simulink model "LQR_6DoF_v4"  (R2022b)
settings: Solver=ode45  StartTime=0.0  StopTime=10  FixedStep=0.01  RelTol=1e-3
undefined symbols (not defined in the file): beta, e0_0, e1_0, e2_0, e3_0, eul0, G0, gamma, gc, geometry, Js, Js0, K_lqrq, m_dry, m_fuel, m_full, m_max, mass, omega0, parameters, pos0, r_cg, rcgs, ref_eul, Tensors, vel0, xq0
libraries: sharedtransform x38, simulink_extras x21, matrix_library x12, sharedutil x4, aerolibpropulsion2 x1
(part 1 of 2)
settings Model: Creator=User  LastModifiedBy=User
settings SolverCC: MaxConsecutiveMinStep=10

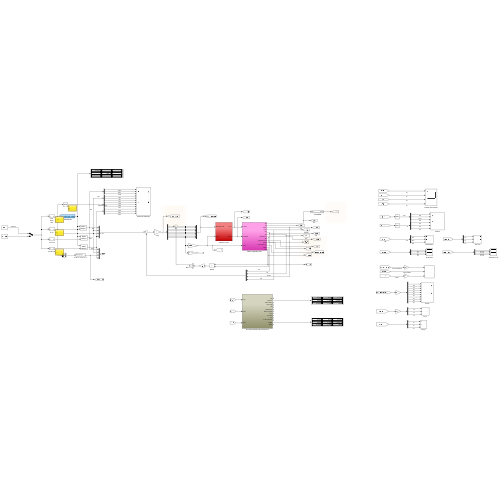
[thumbnail: Simulink's stored preview of the top-level diagram]
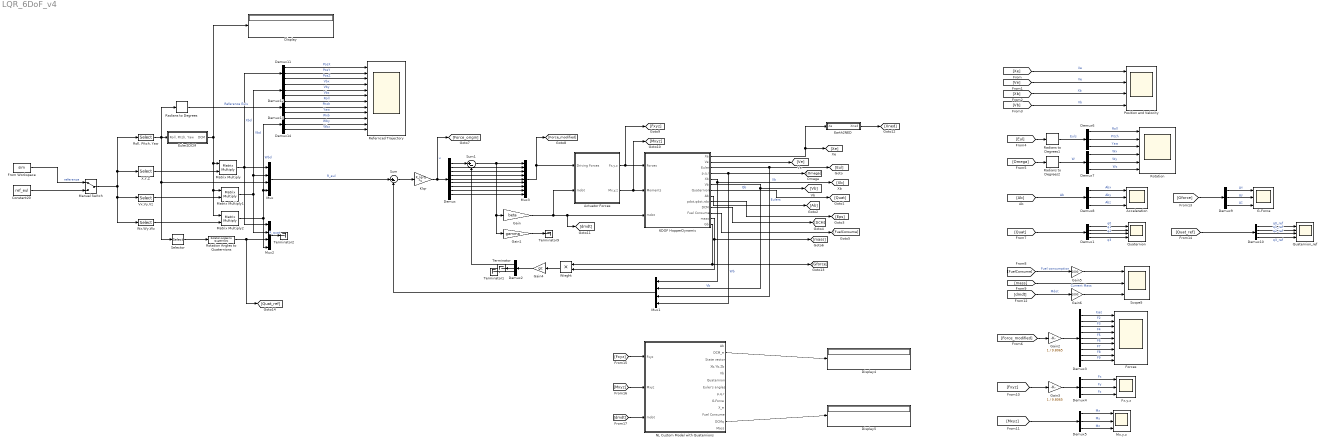
== system LQR_6DoF_v4 ==
  6DOF HopperDynamic : Subsystem
  Acceleration : Scope  NumInputPorts=3
  Actuator Forces : Subsystem
  Constant20 : Constant  Value=ref_eul
  Demux : Demux  Outputs=9
  Demux1 : Demux
  Demux10 : Demux
  Demux{2,4..9,11..14} (11 alike) : Demux  Outputs=3
  Demux3 : Demux  Outputs=9
  Display : Display
  Display4 : Display
  Display5 : Display
  Earth2NED : Subsystem
  Euler2DCM : Subsystem
  Forces : Scope  NumInputPorts=9
  From Workspace : FromWorkspace  VariableName=sim
  Fx,y,z : Scope  NumInputPorts=3
  G-Force : Scope  NumInputPorts=3
  Gain : Gain  Gain=beta
  Gain1 : Gain  Gain=gamma
  Gain2 : Gain  Gain=1 / 9.8065
  Gain3 : Gain  Gain=1 / 9.8065
  Gain4 : Gain  Gain=gc
  Gain5 : Gain  Gain=1000
  Gain6 : Gain  Gain=1000
  Klqr : Gain  Gain=K_lqrq  Multiplication=Matrix(K*u)
  Manual Switch : ManualSwitch
  Matrix Multiply : Product  Multiplication=Matrix(*)
  Matrix Multiply1 : Product  Multiplication=Matrix(*)
  Matrix Multiply2 : Product  Multiplication=Matrix(*)
  Mux : Mux
  Mux1 : Mux
  Mux2 : Mux
  Mux3 : Mux  Inputs=9
  Mx,y,z : Scope  NumInputPorts=3
  NL Custom Model with Quaternions : Subsystem
  Position and Velocity : Scope  NumInputPorts=4
  Quaternion : Scope  NumInputPorts=4
  Quaternion_ref : Scope  NumInputPorts=4
  Radians to Degrees : simulink_extras/Transformations/Radians to Degrees
  Radians to Degrees1 : simulink_extras/Transformations/Radians to Degrees
  Radians to Degrees2 : simulink_extras/Transformations/Radians to Degrees
  Refernced Trajectory : Scope  NumInputPorts=12
  "Roll, Pitch, Yaw" : Selector  InputPortWidth=12  IndexOptions=Index vector (dialog)  Indices=[7:9]  OutputSizes=1
  Rotation : Scope  NumInputPorts=6
  Rotation Angles to Quaternions : sharedtransform/Rotation Angles to Quaternions  rotationOrder=ZYX  aMode=aMode
  Scope5 : Scope  NumInputPorts=3
  Selector : Selector  InputPortWidth=3  IndexOptions=Index vector (dialog)  Indices=[2 3 1]  OutputSizes=1
  Sum : Sum  Inputs=|+-
  Sum1 : Sum  Inputs=|+-
  Terminator{,1..2,9} (4 alike) : Terminator
  Vx,Vy,Vz : Selector  InputPortWidth=12  IndexOptions=Index vector (dialog)  Indices=[4:6]  OutputSizes=1
  Wieght : Product
  Wx,Wy,Wz : Selector  InputPortWidth=12  IndexOptions=Index vector (dialog)  Indices=[10:12]  OutputSizes=1
  X,Y,Z : Selector  InputPortWidth=12  IndexOptions=Index vector (dialog)  Indices=[1:3]  OutputSizes=1
  wires:
  Constant20/1 -> Manual Switch/2
  From Workspace/1 -> Manual Switch/1  "reference"
  "Roll, Pitch, Yaw"/1 -> Radians to Degrees/1, Euler2DCM/1("Roll, Pitch, Yaw"), Selector/1, Mux/3
  Manual Switch/1 -> Wx,Wy,Wz/1, Vx,Vy,Vz/1, X,Y,Z/1, "Roll, Pitch, Yaw"/1
  Euler2DCM/1(DCM) -> Display/1, Matrix Multiply2/1, Matrix Multiply1/1, Matrix Multiply/1
  Klqr/1 -> [Force_origin], Demux/1  "u"
  X,Y,Z/1 -> Matrix Multiply/2
  Vx,Vy,Vz/1 -> Matrix Multiply1/2
  Wx,Wy,Wz/1 -> Matrix Multiply2/2
  Matrix Multiply/1 -> Demux11/1, Mux2/1, Mux/1  "Xbd"
  Actuator Forces/1(Fx,y,z) -> [Fxyz], 6DOF HopperDynamic/1(Forces)
  Actuator Forces/2(Mx,y,z) -> [Mxyz], 6DOF HopperDynamic/2(Moments)
  Demux/1 -> Sum1/1
  Demux/2 -> Mux3/2
  Demux/4 -> Mux3/4
  Demux/6 -> Mux3/6
  Demux/8 -> Mux3/8
  Gain/1 -> Actuator Forces/2(mdot), [dmdt], 6DOF HopperDynamic/3(mdot)
  Gain1/1 -> Terminator9/1
  Matrix Multiply1/1 -> Mux2/2, Demux12/1, Mux/2  "Vbd"
  Matrix Multiply2/1 -> Demux14/1, Mux/4, Mux2/4  "Wbd"
  Radians to Degrees/1 -> Demux13/1  "Reference Euls"
  6DOF HopperDynamic/1(Xe) -> Earth2NED/1(Xe), [Xe]
  6DOF HopperDynamic/2(Ve) -> [Ve]
  6DOF HopperDynamic/3(Euler) -> Mux1/3, [Eul]  "Eulers"
  6DOF HopperDynamic/4(p,q,r) -> Mux1/4, [Omega]  "Wb"
  6DOF HopperDynamic/5(Xb) -> [Xb], Mux1/1  "Xb"
  6DOF HopperDynamic/6(Vb) -> Mux1/2, [Vb]  "Vb"
  6DOF HopperDynamic/7(Quaternion) -> [Quat]  "Qb"
  6DOF HopperDynamic/8(Ab) -> [Ab]
  6DOF HopperDynamic/9(pdot,qdot,rdot) -> [Eps]
  6DOF HopperDynamic/10(DCM) -> [DCM]
  6DOF HopperDynamic/11(Fuel Consume) -> [FuelConsume]
  6DOF HopperDynamic/12(mass) -> Wieght/2, [mass]
  Selector/1 -> Rotation Angles to Quaternions/1
  Rotation Angles to Quaternions/1 -> [Quat_ref], Mux2/3
  Mux/1 -> Sum/1  "R_eul"
  Sum/1 -> Klqr/1
  Mux1/1 -> Sum/2
  [Xe] -> Position and Velocity/1  "Xe"
  [Ve] -> Position and Velocity/2  "Ve"
  [Xb] -> Position and Velocity/3  "Xb"
  [Vb] -> Position and Velocity/4  "Vb"
  [Eul] -> Radians to Degrees1/1
  [Omega] -> Radians to Degrees2/1
  Radians to Degrees1/1 -> Demux6/1  "Euls"
  Radians to Degrees2/1 -> Demux7/1  "W"
  [Ab] -> Demux8/1  "Ab"
  [Quat] -> Demux1/1
  Demux1/1 -> Quaternion/1  "q0"
  Demux1/2 -> Quaternion/2  "q1"
  Demux1/3 -> Quaternion/3  "q2"
  Demux1/4 -> Quaternion/4  "q3"
  [FuelConsume] -> Gain5/1  "Fuel consumption"
  [mass] -> Scope5/2  "Current Mass"
  Demux/3 -> Mux3/3
  Demux/5 -> Mux3/5
  Demux/7 -> Mux3/7
  Demux/9 -> Mux3/9
  Sum1/1 -> Gain1/1, Gain/1, Mux3/1
  Mux3/1 -> [Force_modified], Actuator Forces/1(Driving Forces)
  6DOF HopperDynamic/13(Gb) -> [Gforce], Wieght/1
  Wieght/1 -> Gain4/1
  Demux2/1 -> Sum1/2
  Demux2/2 -> Terminator/1
  Demux2/3 -> Terminator1/1
  [Force_modified] -> Gain2/1
  Gain2/1 -> Demux3/1
  Demux3/1 -> Forces/1  "Fjet"
  Demux3/2 -> Forces/2  "F2"
  Demux3/3 -> Forces/3  "F3"
  Demux3/4 -> Forces/4  "F4"
  Demux3/5 -> Forces/5  "F5"
  Demux3/6 -> Forces/6  "F6"
  Demux3/7 -> Forces/7  "F7"
  Demux3/8 -> Forces/8  "F8"
  Demux3/9 -> Forces/9  "F9"
  [Fxyz] -> Gain3/1
  Gain3/1 -> Demux4/1
  Demux4/1 -> Fx,y,z/1  "Fx"
  Demux4/2 -> Fx,y,z/2  "Fy"
  Demux4/3 -> Fx,y,z/3  "Fz"
  Demux5/2 -> Mx,y,z/2  "My"
  Demux5/1 -> Mx,y,z/1  "Mx"
  [Mxyz] -> Demux5/1
  Demux5/3 -> Mx,y,z/3  "Mz"
  Demux6/2 -> Rotation/2  "Pitch"
  Demux6/1 -> Rotation/1  "Roll"
  Demux6/3 -> Rotation/3  "Yaw"
  Demux7/1 -> Rotation/4  "Wx"
  Demux7/2 -> Rotation/5  "Wy"
  Demux7/3 -> Rotation/6  "Wz"
  Demux8/1 -> Acceleration/1  "Abx"
  Demux8/2 -> Acceleration/2  "Aby"
  Demux8/3 -> Acceleration/3  "Abz"
  [dmdt] -> Gain6/1  "Mdot"
  Earth2NED/1(Xned) -> [Xned]
  [Gforce] -> Demux9/1
  Demux9/1 -> G-Force/1  "gx"
  Demux9/2 -> G-Force/2  "gy"
  Demux9/3 -> G-Force/3  "gz"
  Demux10/2 -> Quaternion_ref/2  "q1_ref"
  Demux10/4 -> Quaternion_ref/4  "q3_ref"
  Demux10/1 -> Quaternion_ref/1  "q0_ref"
  Demux10/3 -> Quaternion_ref/3  "q2_ref"
  [Quat_ref] -> Demux10/1
  [Fxyz] -> NL Custom Model with Quaternions/1(Fxyz)
  [Mxyz] -> NL Custom Model with Quaternions/2(Mxyz)
  [dmdt] -> NL Custom Model with Quaternions/3(mdot)
  NL Custom Model with Quaternions/2(DCM_e) -> Display4/1
  NL Custom Model with Quaternions/12(DCMq) -> Display5/1
  Mux2/1 -> Terminator2/1  "R_quat"
  Gain4/1 -> Demux2/1
  Gain5/1 -> Scope5/1
  Gain6/1 -> Scope5/3
  Demux11/1 -> Refernced Trajectory/1  "PosX"
  Demux11/2 -> Refernced Trajectory/2  "PosY"
  Demux11/3 -> Refernced Trajectory/3  "PosZ"
  Demux12/1 -> Refernced Trajectory/4  "Vbx"
  Demux12/2 -> Refernced Trajectory/5  "Vby"
  Demux12/3 -> Refernced Trajectory/6  "Vbz"
  Demux13/1 -> Refernced Trajectory/7  "Roll"
  Demux13/2 -> Refernced Trajectory/8  "Pitch"
  Demux13/3 -> Refernced Trajectory/9  "Yaw"
  Demux14/1 -> Refernced Trajectory/10  "Wxb"
  Demux14/2 -> Refernced Trajectory/11  "Wby"
  Demux14/3 -> Refernced Trajectory/12  "Wbz"

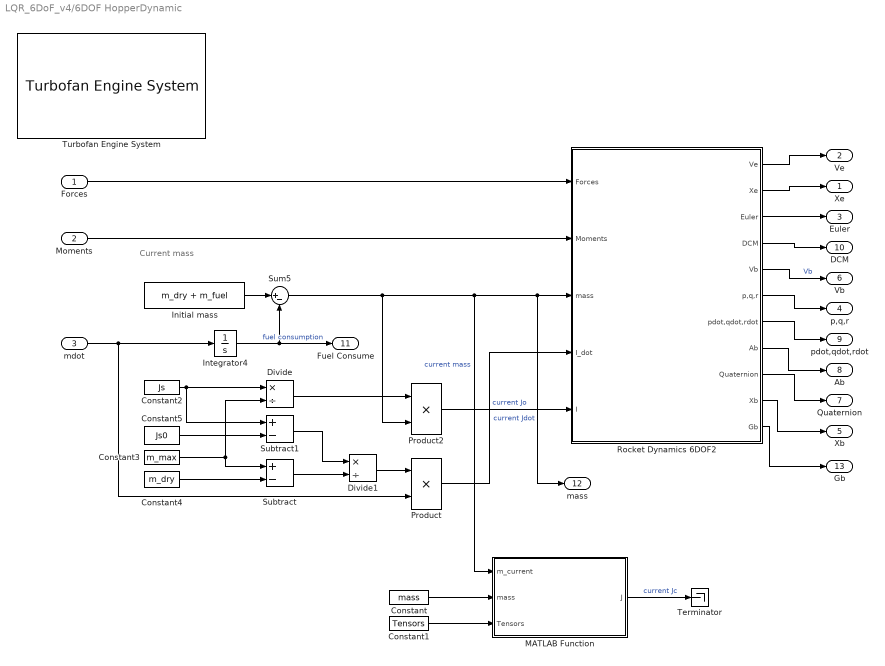
== system LQR_6DoF_v4/6DOF HopperDynamic ==
  note: Current mass
  Forces : Inport
  Moments : Inport  Port=2
  mdot : Inport  Port=3
  Constant : Constant  Value=mass
  Constant1 : Constant  Value=Tensors
  Constant2 : Constant  Value=Js
  Constant3 : Constant  Value=m_max
  Constant4 : Constant  Value=m_dry
  Constant5 : Constant  Value=Js0
  Divide : Product  Inputs=*/
  Divide1 : Product  Inputs=*/
  Initial mass : Constant  Value=m_dry + m_fuel
  Integrator4 : Integrator
  MATLAB Function : MATLAB Function  TreatAsAtomicUnit=on
  Product : Product  SaturateOnIntegerOverflow=on  OutDataTypeStr=Inherit: Same as first input
  Product2 : Product  SaturateOnIntegerOverflow=on  OutDataTypeStr=Inherit: Same as first input
  Rocket Dynamics 6DOF2 : Subsystem  mask(6DOF EoM (Body Axis)){xme_0=pos0', Vm_0=vel0', eul_0=eul0', pm_0=omega0', k_quat=1.0, xme_statename='', Vm_statename='', quat_statename='', pm_statename=''}
      mask prompts: xme_0 "Initial position in inertial axes [Xe,Ye,Ze]:"; Vm_0 "Initial velocity in body axes [U,v,w]:"; eul_0 "Initial Euler orientation [roll, pitch, yaw]:"; pm_0 "Initial body rotation rates [p,q,r]:"; k_quat "Gain for quaternion normalization:"; xme_statename "Position: e.g., {'Xe', 'Ye', 'Ze'}"; Vm_statename "Velocity: e.g., {'U', 'v', 'w'}"; quat_statename "Quaternion vector: e.g., {'qr', 'qi', 'qj', 'qk'}"; pm_statename "Body rotation rates: e.g., {'p', 'q', 'r'}"
      mask help: Integrate the six-degress-of-freedom equations of motion in body axes
      mask DialogControl Container8 Prompt: Main
      mask DialogControl Container9 Prompt: State Attributes
      mask DialogControl Container10 Prompt: State Names
      mask Display:
      | port_label('input',1,'F_{xyz}(N)','texmode','on');
      | port_label('input',2,'M_{xyz}(N\cdotm)','texmode','on');
      | port_label('input',3,'m (kg)','texmode','on');
      | port_label('input',4,'dI/dt (kg\cdotm^2/s)','texmode','on');
      | port_label('input',5,'I (kg\cdotm^2)','texmode','on');
      | port_label('output',1,'V_e (m/s)','texmode','on');
      | port_label('output',2,'X_e (m)','texmode','on');
      | port_label('output',3,'\phi \theta \psi (rad)','texmode','on');
      | port_label('output',4,'DCM_{be}','texmode','on');
      | port_label('output',5,'V_b (m/s)','texmode','on');
      | port_label('output',6,'\omega_b (rad/s)','texmode','on');
      | port_label('output',7,'d\omega_b/dt (rad/s^2)','texmode','on');
      | port_label('output',8,'A_{bb} (m/s^2)','texmode','on');
  Subtract : Sum  Inputs=+-
  Subtract1 : Sum  Inputs=+-
  Sum5 : Sum  Inputs=|+-
  Terminator : Terminator
  Turbofan Engine System : aerolibpropulsion2/Turbofan Engine System  units=Metric (MKS)  ic_source=Internal  IC=0  Fmax=45000  tau=1  SFC=0.35  Nt=0.9
  Xe : Outport
  Ve : Outport  Port=2
  Euler : Outport  Port=3
  p,q,r : Outport  Port=4
  Xb : Outport  Port=5
  Vb : Outport  Port=6
  Quaternion : Outport  Port=7
  Ab : Outport  Port=8
  pdot,qdot,rdot : Outport  Port=9
  DCM : Outport  Port=10
  Fuel Consume : Outport  Port=11
  mass : Outport  Port=12
  Gb : Outport  Port=13
  wires:
  Rocket Dynamics 6DOF2/6(p,q,r) -> p,q,r/1
  Divide/1 -> Product2/1
  Integrator4/1 -> Fuel Consume/1, Sum5/2  "fuel consumption"
  Constant3/1 -> Divide/2, Subtract/1
  Product2/1 -> Rocket Dynamics 6DOF2/5(I)  "current Jo"
  Rocket Dynamics 6DOF2/4(DCM) -> DCM/1
  Constant5/1 -> Subtract1/2
  Rocket Dynamics 6DOF2/5(Vb) -> Vb/1  "Vb"
  Subtract1/1 -> Divide1/1
  Divide1/1 -> Product/1
  mdot/1 -> Product/2, Integrator4/1
  Constant4/1 -> Subtract/2
  Sum5/1 -> Product2/2, MATLAB Function/1(m_current), mass/1, Rocket Dynamics 6DOF2/3(mass)  "current mass"
  Subtract/1 -> Divide1/2
  Constant2/1 -> Divide/1, Subtract1/1
  Rocket Dynamics 6DOF2/2(Xe) -> Xe/1
  Initial mass/1 -> Sum5/1
  Product/1 -> Rocket Dynamics 6DOF2/4(I_dot)  "current Jdot"
  Rocket Dynamics 6DOF2/8(Ab) -> Ab/1
  Rocket Dynamics 6DOF2/1(Ve) -> Ve/1
  Forces/1 -> Rocket Dynamics 6DOF2/1(Forces)
  Rocket Dynamics 6DOF2/3(Euler) -> Euler/1
  Rocket Dynamics 6DOF2/9(Quaternion) -> Quaternion/1
  Moments/1 -> Rocket Dynamics 6DOF2/2(Moments)
  Rocket Dynamics 6DOF2/7(pdot,qdot,rdot) -> pdot,qdot,rdot/1
  Rocket Dynamics 6DOF2/10(Xb) -> Xb/1
  Rocket Dynamics 6DOF2/11(Gb) -> Gb/1
  Constant/1 -> MATLAB Function/2(mass)
  Constant1/1 -> MATLAB Function/3(Tensors)
  MATLAB Function/1(J) -> Terminator/1  "current Jc"

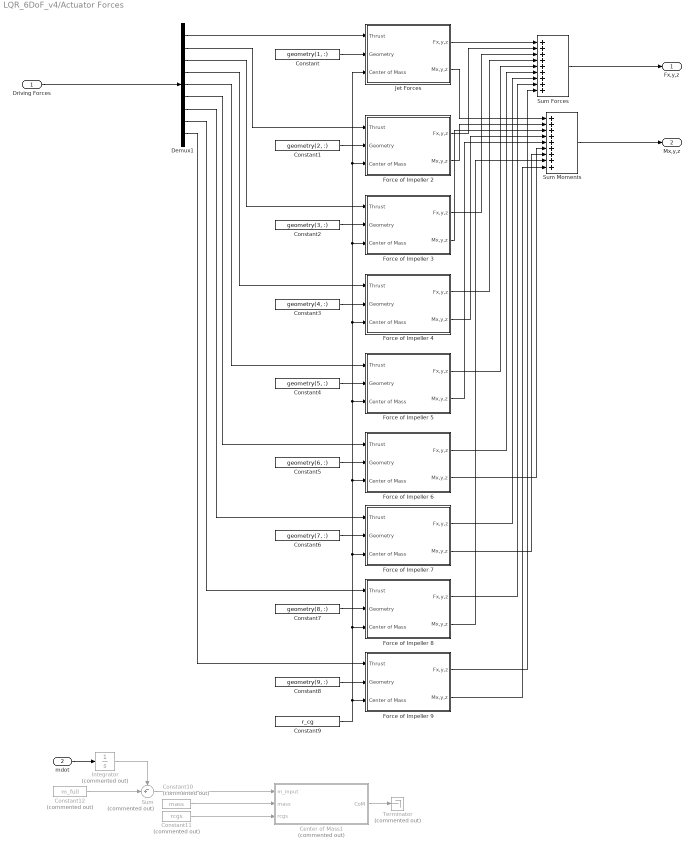
== system LQR_6DoF_v4/Actuator Forces ==
  Driving Forces : Inport
  mdot : Inport  Port=2
  Center of Mass1 : MATLAB Function  Commented=on  TreatAsAtomicUnit=on
  Constant : Constant  Value=geometry(1, :)
  Constant1 : Constant  Value=geometry(2, :)
  Constant10 : Constant  Commented=on  Value=mass
  Constant11 : Constant  Commented=on  Value=rcgs
  Constant12 : Constant  Commented=on  Value=m_full
  Constant2 : Constant  Value=geometry(3, :)
  Constant3 : Constant  Value=geometry(4, :)
  Constant4 : Constant  Value=geometry(5, :)
  Constant5 : Constant  Value=geometry(6, :)
  Constant6 : Constant  Value=geometry(7, :)
  Constant7 : Constant  Value=geometry(8, :)
  Constant8 : Constant  Value=geometry(9, :)
  Constant9 : Constant  Value=r_cg
  Demux1 : Demux  Outputs=9
  Force of Impeller 2 : Subsystem
  Force of Impeller 3 : Subsystem
  Force of Impeller 4 : Subsystem
  Force of Impeller 5 : Subsystem
  Force of Impeller 6 : Subsystem
  Force of Impeller 7 : Subsystem
  Force of Impeller 8 : Subsystem
  Force of Impeller 9 : Subsystem
  Integrator : Integrator  Commented=on
  Jet Forces : Subsystem
  Sum : Sum  Commented=on  Inputs=-+|
  Sum Forces : Sum  Inputs=+++++++++
  Sum Moments : Sum  Inputs=+++++++++
  Terminator : Terminator  Commented=on
  Fx,y,z : Outport
  Mx,y,z : Outport  Port=2
  wires:
  Force of Impeller 8/1(Fx,y,z) -> Sum Forces/8
  Constant9/1 -> Jet Forces/3(Center of Mass), Force of Impeller 2/3(Center of Mass), Force of Impeller 3/3(Center of Mass), Force of Impeller 4/3(Center of Mass), Force of Impeller 5/3(Center of Mass), Force of Impeller 6/3(Center of Mass), Force of Impeller 7/3(Center of Mass), Force of Impeller 8/3(Center of Mass), Force of Impeller 9/3(Center of Mass)
  Demux1/4 -> Force of Impeller 4/1(Thrust)
  Force of Impeller 9/1(Fx,y,z) -> Sum Forces/9
  Demux1/9 -> Force of Impeller 9/1(Thrust)
  Force of Impeller 5/2(Mx,y,z) -> Sum Moments/5
  Constant1/1 -> Force of Impeller 2/2(Geometry)
  Sum Forces/1 -> Fx,y,z/1
  Force of Impeller 7/2(Mx,y,z) -> Sum Moments/7
  Demux1/6 -> Force of Impeller 6/1(Thrust)
  Demux1/1 -> Jet Forces/1(Thrust)
  Force of Impeller 6/1(Fx,y,z) -> Sum Forces/6
  Constant7/1 -> Force of Impeller 8/2(Geometry)
  Demux1/3 -> Force of Impeller 3/1(Thrust)
  Sum Moments/1 -> Mx,y,z/1
  Jet Forces/2(Mx,y,z) -> Sum Moments/1
  Jet Forces/1(Fx,y,z) -> Sum Forces/1
  Force of Impeller 8/2(Mx,y,z) -> Sum Moments/8
  Force of Impeller 6/2(Mx,y,z) -> Sum Moments/6
  Force of Impeller 3/1(Fx,y,z) -> Sum Forces/3
  Demux1/5 -> Force of Impeller 5/1(Thrust)
  Force of Impeller 4/1(Fx,y,z) -> Sum Forces/4
  Force of Impeller 2/2(Mx,y,z) -> Sum Moments/2
  Force of Impeller 4/2(Mx,y,z) -> Sum Moments/4
  Force of Impeller 3/2(Mx,y,z) -> Sum Moments/3
  Force of Impeller 5/1(Fx,y,z) -> Sum Forces/5
  Constant3/1 -> Force of Impeller 4/2(Geometry)
  Force of Impeller 7/1(Fx,y,z) -> Sum Forces/7
  Constant6/1 -> Force of Impeller 7/2(Geometry)
  Force of Impeller 9/2(Mx,y,z) -> Sum Moments/9
  Demux1/7 -> Force of Impeller 7/1(Thrust)
  Constant5/1 -> Force of Impeller 6/2(Geometry)
  Constant8/1 -> Force of Impeller 9/2(Geometry)
  Constant4/1 -> Force of Impeller 5/2(Geometry)
  Demux1/2 -> Force of Impeller 2/1(Thrust)
  Force of Impeller 2/1(Fx,y,z) -> Sum Forces/2
  Demux1/8 -> Force of Impeller 8/1(Thrust)
  Driving Forces/1 -> Demux1/1
  Constant/1 -> Jet Forces/2(Geometry)
  Constant2/1 -> Force of Impeller 3/2(Geometry)
  Constant10/1 -> Center of Mass1/2(mass)
  Constant11/1 -> Center of Mass1/3(rcgs)
  mdot/1 -> Integrator/1
  Constant12/1 -> Sum/2
  Integrator/1 -> Sum/1
  Sum/1 -> Center of Mass1/1(m_input)
  Center of Mass1/1(CoM) -> Terminator/1

== system LQR_6DoF_v4/Earth2NED ==
  Xe : Inport
  Constant10 : Constant  Value=deg2rad([90, 0, 0])
  Euler2DCM : Subsystem
  Matrix Multiply : Product  Multiplication=Matrix(*)
  Xned : Outport
  wires:
  Euler2DCM/1(DCM) -> Matrix Multiply/1
  Constant10/1 -> Euler2DCM/1("Roll, Pitch, Yaw")
  Matrix Multiply/1 -> Xned/1
  Xe/1 -> Matrix Multiply/2

== system LQR_6DoF_v4/Euler2DCM ==
  "Roll, Pitch, Yaw" : Inport
  "Pitch, Yaw, Roll" : Selector  InputPortWidth=3  IndexOptions=Index vector (dialog)  Indices=[2 3 1]  OutputSizes=1
  Quaternions to Direction Cosine Matrix : sharedtransform/Quaternions to  Direction Cosine Matrix  aMode=aMode
  Rotation Angles to Quaternions : sharedtransform/Rotation Angles to Quaternions  rotationOrder=ZYX  aMode=aMode
  DCM : Outport
  wires:
  "Roll, Pitch, Yaw"/1 -> "Pitch, Yaw, Roll"/1
  "Pitch, Yaw, Roll"/1 -> Rotation Angles to Quaternions/1
  Rotation Angles to Quaternions/1 -> Quaternions to Direction Cosine Matrix/1
  Quaternions to Direction Cosine Matrix/1 -> DCM/1

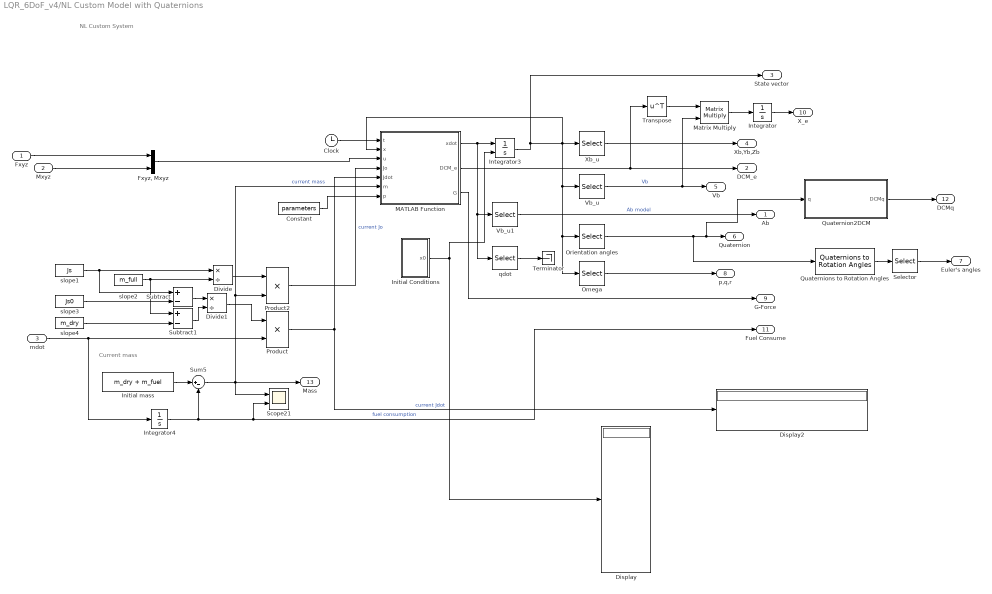
== system LQR_6DoF_v4/NL Custom Model with Quaternions ==
  note: NL Custom System
  note: Current mass
  Fxyz : Inport
  Mxyz : Inport  Port=2
  mdot : Inport  Port=3
  Clock : Clock
  Constant : Constant  Value=parameters
  Display : Display
  Display2 : Display
  Divide : Product  Inputs=*/
  Divide1 : Product  Inputs=*/
  "Fxyz, Mxyz" : Mux  Inputs=2
  Initial Conditions : Subsystem
  Initial mass : Constant  Value=m_dry + m_fuel
  Integrator : Integrator  InitialCondition=[0; 0; 0]
  Integrator3 : Integrator  InitialConditionSource=external  InitialCondition=xq0'
  Integrator4 : Integrator
  MATLAB Function : MATLAB Function  TreatAsAtomicUnit=on
  Matrix Multiply : Product  Multiplication=Matrix(*)
  Omega : Selector  InputPortWidth=13  IndexOptions=Index vector (dialog)  Indices=11:13  OutputSizes=1
  Orientation angles : Selector  InputPortWidth=13  IndexOptions=Index vector (dialog)  Indices=7:10  OutputSizes=1
  Product : Product  SaturateOnIntegerOverflow=on  OutDataTypeStr=Inherit: Same as first input
  Product2 : Product  SaturateOnIntegerOverflow=on  OutDataTypeStr=Inherit: Same as first input
  Quaternion2DCM : Subsystem
  Quaternions to Rotation Angles : sharedtransform/Quaternions to Rotation Angles  rotationOrder=ZYX  aMode=aMode
  Scope21 : Scope  NumInputPorts=2
  Selector : Selector  InputPortWidth=3  IndexOptions=Index vector (dialog)  Indices=[3 1 2]  OutputSizes=1
  Subtract : Sum  Inputs=+-
  Subtract1 : Sum  Inputs=+-
  Sum5 : Sum  Inputs=|+-
  Terminator : Terminator
  Transpose : Math  Operator=transpose
  Vb_u : Selector  InputPortWidth=13  IndexOptions=Index vector (dialog)  Indices=4:6  OutputSizes=1
  Vb_u1 : Selector  InputPortWidth=13  IndexOptions=Index vector (dialog)  Indices=4:6  OutputSizes=1
  Xb_u : Selector  InputPortWidth=13  IndexOptions=Index vector (dialog)  Indices=1:3  OutputSizes=1
  qdot : Selector  InputPortWidth=13  IndexOptions=Index vector (dialog)  Indices=7:10  OutputSizes=1
  slope1 : Constant  Value=Js  OutDataTypeStr=Inherit: Inherit via back propagation
  slope2 : Constant  Value=m_full  OutDataTypeStr=Inherit: Inherit via back propagation
  slope3 : Constant  Value=Js0  OutDataTypeStr=Inherit: Inherit via back propagation
  slope4 : Constant  Value=m_dry  OutDataTypeStr=Inherit: Inherit via back propagation
  Ab : Outport
  DCM_e : Outport  Port=2
  State vector : Outport  Port=3
  Xb,Yb,Zb : Outport  Port=4
  Vb : Outport  Port=5
  Quaternion : Outport  Port=6
  Euler's angles : Outport  Port=7
  p,q,r : Outport  Port=8
  G-Force : Outport  Port=9
  X_e : Outport  Port=10
  Fuel Consume : Outport  Port=11
  DCMq : Outport  Port=12
  Mass : Outport  Port=13
  wires:
  Integrator3/1 -> State vector/1, MATLAB Function/2(x), Omega/1, Orientation angles/1, Vb_u/1, Xb_u/1
  mdot/1 -> Product/2, Integrator4/1
  MATLAB Function/3(G) -> G-Force/1
  Product/1 -> Display2/1, MATLAB Function/5(Jdot)  "current Jdot"
  Integrator4/1 -> Sum5/2, Scope21/2, Fuel Consume/1  "fuel consumption"
  Vb_u1/1 -> Ab/1  "Ab model"
  MATLAB Function/2(DCM_e) -> Transpose/1, DCM_e/1
  slope1/1 -> Subtract/1, Divide/1
  Sum5/1 -> Mass/1, MATLAB Function/6(m), Product2/2, Scope21/1  "current mass"
  Product2/1 -> MATLAB Function/4(Jo)  "current Jo"
  Clock/1 -> MATLAB Function/1(t)
  MATLAB Function/1(xdot) -> qdot/1, Vb_u1/1, Integrator3/1
  "Fxyz, Mxyz"/1 -> MATLAB Function/3(u)
  Fxyz/1 -> "Fxyz, Mxyz"/1
  Initial mass/1 -> Sum5/1
  Divide1/1 -> Product/1
  Xb_u/1 -> Xb,Yb,Zb/1
  Vb_u/1 -> Matrix Multiply/2, Vb/1  "Vb"
  Omega/1 -> p,q,r/1
  Mxyz/1 -> "Fxyz, Mxyz"/2
  Orientation angles/1 -> Quaternions to Rotation Angles/1, Quaternion2DCM/1(q), Quaternion/1
  Matrix Multiply/1 -> Integrator/1
  Quaternions to Rotation Angles/1 -> Selector/1
  Selector/1 -> Euler's angles/1
  qdot/1 -> Terminator/1
  slope2/1 -> Subtract1/1, Divide/2
  Divide/1 -> Product2/1
  slope3/1 -> Subtract/2
  slope4/1 -> Subtract1/2
  Subtract/1 -> Divide1/1
  Subtract1/1 -> Divide1/2
  Initial Conditions/1(x0) -> Integrator3/2, Display/1
  Quaternion2DCM/1(DCMq) -> DCMq/1
  Constant/1 -> MATLAB Function/7(p)
  Transpose/1 -> Matrix Multiply/1
  Integrator/1 -> X_e/1

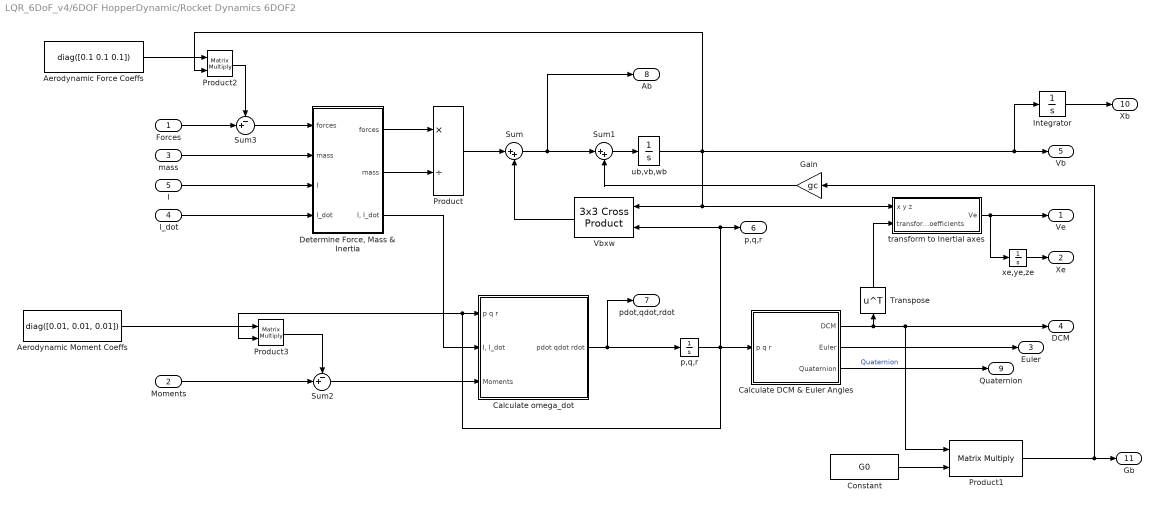
== system LQR_6DoF_v4/6DOF HopperDynamic/Rocket Dynamics 6DOF2 ==
  Forces : Inport  Unit=N  PortDimensions=3
  Moments : Inport  Port=2  Unit=N*m  PortDimensions=3
  mass : Inport  Port=3  Unit=kg
  I_dot : Inport  Port=4  Unit=kg*m^2/s  PortDimensions=[3 3]
  I : Inport  Port=5  Unit=kg*m^2  PortDimensions=[3 3]
  Aerodynamic Force Coeffs : Constant  Value=diag([0.1 0.1 0.1])
  Aerodynamic Moment Coeffs : Constant  Value=diag([0.01, 0.01, 0.01])
  Calculate DCM & Euler Angles : Subsystem
  Calculate omega_dot : Subsystem
  Constant : Constant  Value=G0
  "Determine Force, Mass & Inertia" : Subsystem
  Gain : Gain  Gain=gc
  Integrator : Integrator
  Product : Product  Inputs=*/  SaturateOnIntegerOverflow=on  OutDataTypeStr=Inherit: Same as first input
  Product1 : Product  Multiplication=Matrix(*)
  Product2 : Product  Multiplication=Matrix(*)
  Product3 : Product  Multiplication=Matrix(*)
  Sum : Sum  Inputs=|++  SaturateOnIntegerOverflow=on
  Sum1 : Sum  Inputs=|++
  Sum2 : Sum  Inputs=-+|
  Sum3 : Sum  Inputs=-+|
  Transpose : Math  Operator=transpose  SignedPower=on
  Vbxw : sharedutil/3x3 Cross Product  aMode=aMode
  "p,q,r " : Integrator  InitialCondition=pm_0  ContinuousStateAttributes=pm_statename
  transform to Inertial axes : Subsystem
  ub,vb,wb : Integrator  InitialCondition=Vm_0  ContinuousStateAttributes=Vm_statename
  xe,ye,ze : Integrator  InitialCondition=xme_0  ContinuousStateAttributes=xme_statename
  Ve : Outport  Unit=m/s  VectorParamsAs1DForOutWhenUnconnected=off
  Xe : Outport  Port=2  Unit=m  VectorParamsAs1DForOutWhenUnconnected=off
  Euler : Outport  Port=3  Unit=rad  VectorParamsAs1DForOutWhenUnconnected=off
  DCM : Outport  Port=4  Unit=1  VectorParamsAs1DForOutWhenUnconnected=off
  Vb : Outport  Port=5  Unit=m/s  VectorParamsAs1DForOutWhenUnconnected=off
  p,q,r : Outport  Port=6  Unit=rad/s  VectorParamsAs1DForOutWhenUnconnected=off
  pdot,qdot,rdot : Outport  Port=7  Unit=rad/s^2  VectorParamsAs1DForOutWhenUnconnected=off
  Ab : Outport  Port=8  Unit=m/s^2  VectorParamsAs1DForOutWhenUnconnected=off
  Quaternion : Outport  Port=9
  Xb : Outport  Port=10
  Gb : Outport  Port=11
  wires:
  Forces/1 -> Sum3/2
  mass/1 -> "Determine Force, Mass & Inertia"/2("mass ")
  I/1 -> "Determine Force, Mass & Inertia"/3(I)
  I_dot/1 -> "Determine Force, Mass & Inertia"/4(I_dot)
  "Determine Force, Mass & Inertia"/1("forces ") -> Product/1
  "Determine Force, Mass & Inertia"/2(mass) -> Product/2
  Product/1 -> Sum/1
  Sum/1 -> Ab/1, Sum1/1
  Vbxw/1 -> Sum/2
  "Determine Force, Mass & Inertia"/3("I, I_dot ") -> Calculate omega_dot/2("I, I_dot")
  ub,vb,wb/1 -> Product2/2, Integrator/1, Vb/1, transform to Inertial axes/1(x y z), Vbxw/1
  Calculate omega_dot/1(pdot qdot rdot) -> "p,q,r "/1, pdot,qdot,rdot/1
  xe,ye,ze/1 -> Xe/1
  transform to Inertial axes/1(Ve) -> xe,ye,ze/1, Ve/1
  "p,q,r "/1 -> Calculate DCM & Euler Angles/1(p q r), Vbxw/2, p,q,r/1, Product3/2, Calculate omega_dot/1(p q r)
  Moments/1 -> Sum2/2
  Calculate DCM & Euler Angles/1(DCM) -> Product1/1, DCM/1, Transpose/1
  Calculate DCM & Euler Angles/2(Euler) -> Euler/1
  Transpose/1 -> transform to Inertial axes/2(transform coefficients)
  Calculate DCM & Euler Angles/3(Quaternion) -> Quaternion/1  "Quaternion"
  Constant/1 -> Product1/2
  Product1/1 -> Gb/1, Gain/1
  Sum1/1 -> ub,vb,wb/1
  Sum2/1 -> Calculate omega_dot/3(Moments)
  Sum3/1 -> "Determine Force, Mass & Inertia"/1(forces)
  Aerodynamic Force Coeffs/1 -> Product2/1
  Product2/1 -> Sum3/1
  Aerodynamic Moment Coeffs/1 -> Product3/1
  Product3/1 -> Sum2/1
  Integrator/1 -> Xb/1
  Gain/1 -> Sum1/2

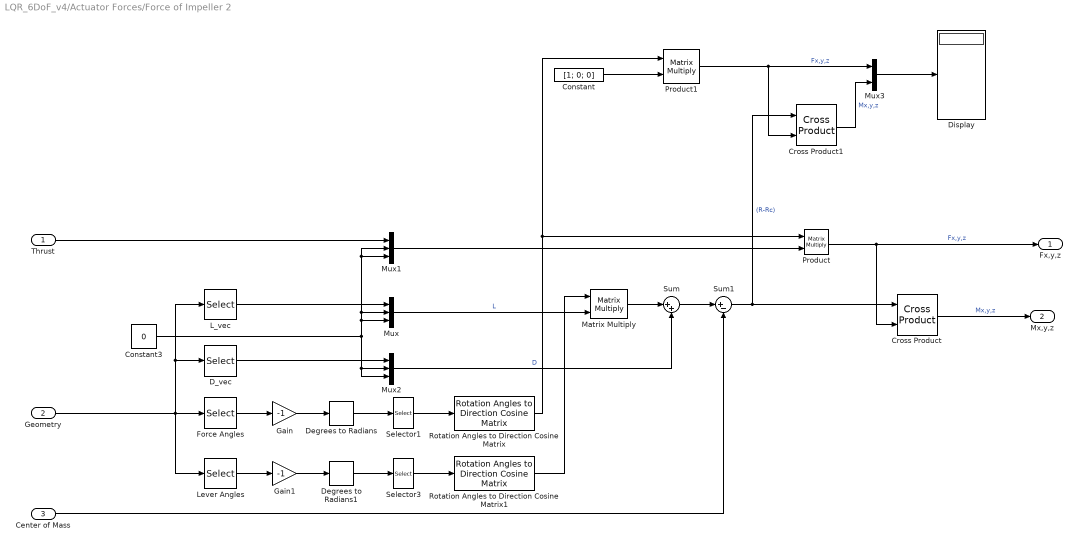
== system LQR_6DoF_v4/Actuator Forces/Force of Impeller 2 ==
  Thrust : Inport
  Geometry : Inport  Port=2
  Center of Mass : Inport  Port=3
  Constant : Constant  Value=[1; 0; 0]
  Constant3 : Constant  Value=0
  Cross Product : matrix_library/Cross Product
  Cross Product1 : matrix_library/Cross Product
  D_vec : Selector  InputPortWidth=9  IndexOptions=Index vector (dialog)  Indices=[2]  OutputSizes=1
  Degrees to Radians : simulink_extras/Transformations/Degrees to Radians
  Degrees to Radians1 : simulink_extras/Transformations/Degrees to Radians
  Display : Display
  Force Angles : Selector  InputPortWidth=9  IndexOptions=Index vector (dialog)  Indices=[4:6]  OutputSizes=1
  Gain : Gain  Gain=-1
  Gain1 : Gain  Gain=-1
  L_vec : Selector  InputPortWidth=9  IndexOptions=Index vector (dialog)  Indices=[1]  OutputSizes=1
  Lever Angles : Selector  InputPortWidth=9  IndexOptions=Index vector (dialog)  Indices=[7:9]  OutputSizes=1
  Matrix Multiply : Product  Multiplication=Matrix(*)
  Mux : Mux  Inputs=3
  Mux1 : Mux  Inputs=3
  Mux2 : Mux  Inputs=3
  Mux3 : Mux  Inputs=2
  Product : Product  Multiplication=Matrix(*)
  Product1 : Product  Multiplication=Matrix(*)
  Rotation Angles to Direction Cosine Matrix : sharedtransform/Rotation Angles to Direction Cosine Matrix  rotationOrder=ZYX  aMode=aMode
  Rotation Angles to Direction Cosine Matrix1 : sharedtransform/Rotation Angles to Direction Cosine Matrix  rotationOrder=ZYX  aMode=aMode
  Selector1 : Selector  InputPortWidth=3  IndexOptions=Index vector (dialog)  Indices=[2 3 1]  OutputSizes=1
  Selector3 : Selector  InputPortWidth=3  IndexOptions=Index vector (dialog)  Indices=[2 3 1]  OutputSizes=1
  Sum : Sum  Inputs=|++
  Sum1 : Sum  Inputs=|+-
  Fx,y,z : Outport
  Mx,y,z : Outport  Port=2
  wires:
  Product/1 -> Fx,y,z/1, Cross Product/2  "Fx,y,z"
  Rotation Angles to Direction Cosine Matrix1/1 -> Matrix Multiply/1
  Constant3/1 -> Mux2/3, Mux2/2, Mux/3, Mux1/3, Mux1/2, Mux/2
  Degrees to Radians/1 -> Selector1/1
  Mux2/1 -> Sum/2  "D"
  Cross Product/1 -> Mx,y,z/1  "Mx,y,z"
  Geometry/1 -> Force Angles/1, Lever Angles/1, D_vec/1, L_vec/1
  Sum/1 -> Sum1/1
  Degrees to Radians1/1 -> Selector3/1
  L_vec/1 -> Mux/1
  D_vec/1 -> Mux2/1
  Selector3/1 -> Rotation Angles to Direction Cosine Matrix1/1
  Force Angles/1 -> Gain/1
  Selector1/1 -> Rotation Angles to Direction Cosine Matrix/1
  Mux/1 -> Matrix Multiply/2  "L"
  Matrix Multiply/1 -> Sum/1
  Lever Angles/1 -> Gain1/1
  Thrust/1 -> Mux1/1
  Center of Mass/1 -> Sum1/2
  Gain1/1 -> Degrees to Radians1/1
  Gain/1 -> Degrees to Radians/1
  Mux1/1 -> Product/2
  Sum1/1 -> Cross Product1/1, Cross Product/1  "(R-Rc)"
  Constant/1 -> Product1/2
  Rotation Angles to Direction Cosine Matrix/1 -> Product/1, Product1/1
  Mux3/1 -> Display/1
  Product1/1 -> Cross Product1/2, Mux3/1  "Fx,y,z"
  Cross Product1/1 -> Mux3/2  "Mx,y,z"

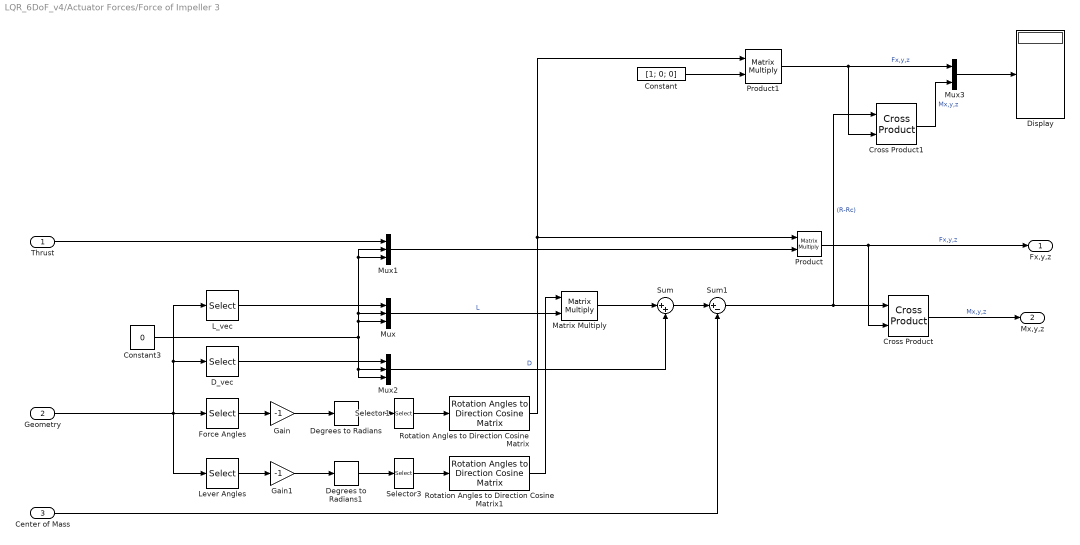
== system LQR_6DoF_v4/Actuator Forces/Force of Impeller 3 ==
  Thrust : Inport
  Geometry : Inport  Port=2
  Center of Mass : Inport  Port=3
  Constant : Constant  Value=[1; 0; 0]
  Constant3 : Constant  Value=0
  Cross Product : matrix_library/Cross Product
  Cross Product1 : matrix_library/Cross Product
  D_vec : Selector  InputPortWidth=9  IndexOptions=Index vector (dialog)  Indices=[2]  OutputSizes=1
  Degrees to Radians : simulink_extras/Transformations/Degrees to Radians
  Degrees to Radians1 : simulink_extras/Transformations/Degrees to Radians
  Display : Display
  Force Angles : Selector  InputPortWidth=9  IndexOptions=Index vector (dialog)  Indices=[4:6]  OutputSizes=1
  Gain : Gain  Gain=-1
  Gain1 : Gain  Gain=-1
  L_vec : Selector  InputPortWidth=9  IndexOptions=Index vector (dialog)  Indices=[1]  OutputSizes=1
  Lever Angles : Selector  InputPortWidth=9  IndexOptions=Index vector (dialog)  Indices=[7:9]  OutputSizes=1
  Matrix Multiply : Product  Multiplication=Matrix(*)
  Mux : Mux  Inputs=3
  Mux1 : Mux  Inputs=3
  Mux2 : Mux  Inputs=3
  Mux3 : Mux  Inputs=2
  Product : Product  Multiplication=Matrix(*)
  Product1 : Product  Multiplication=Matrix(*)
  Rotation Angles to Direction Cosine Matrix : sharedtransform/Rotation Angles to Direction Cosine Matrix  rotationOrder=ZYX  aMode=aMode
  Rotation Angles to Direction Cosine Matrix1 : sharedtransform/Rotation Angles to Direction Cosine Matrix  rotationOrder=ZYX  aMode=aMode
  Selector1 : Selector  InputPortWidth=3  IndexOptions=Index vector (dialog)  Indices=[2 3 1]  OutputSizes=1
  Selector3 : Selector  InputPortWidth=3  IndexOptions=Index vector (dialog)  Indices=[2 3 1]  OutputSizes=1
  Sum : Sum  Inputs=|++
  Sum1 : Sum  Inputs=|+-
  Fx,y,z : Outport
  Mx,y,z : Outport  Port=2
  wires:
  Product/1 -> Fx,y,z/1, Cross Product/2  "Fx,y,z"
  Rotation Angles to Direction Cosine Matrix1/1 -> Matrix Multiply/1
  Constant3/1 -> Mux2/3, Mux2/2, Mux/3, Mux1/3, Mux1/2, Mux/2
  Degrees to Radians/1 -> Selector1/1
  Mux2/1 -> Sum/2  "D"
  Cross Product/1 -> Mx,y,z/1  "Mx,y,z"
  Mux1/1 -> Product/2
  Geometry/1 -> Force Angles/1, Lever Angles/1, D_vec/1, L_vec/1
  Sum/1 -> Sum1/1
  Degrees to Radians1/1 -> Selector3/1
  L_vec/1 -> Mux/1
  D_vec/1 -> Mux2/1
  Selector3/1 -> Rotation Angles to Direction Cosine Matrix1/1
  Force Angles/1 -> Gain/1
  Selector1/1 -> Rotation Angles to Direction Cosine Matrix/1
  Mux/1 -> Matrix Multiply/2  "L"
  Matrix Multiply/1 -> Sum/1
  Lever Angles/1 -> Gain1/1
  Thrust/1 -> Mux1/1
  Center of Mass/1 -> Sum1/2
  Gain/1 -> Degrees to Radians/1
  Gain1/1 -> Degrees to Radians1/1
  Rotation Angles to Direction Cosine Matrix/1 -> Product/1, Product1/1
  Constant/1 -> Product1/2
  Mux3/1 -> Display/1
  Sum1/1 -> Cross Product1/1, Cross Product/1  "(R-Rc)"
  Product1/1 -> Cross Product1/2, Mux3/1  "Fx,y,z"
  Cross Product1/1 -> Mux3/2  "Mx,y,z"

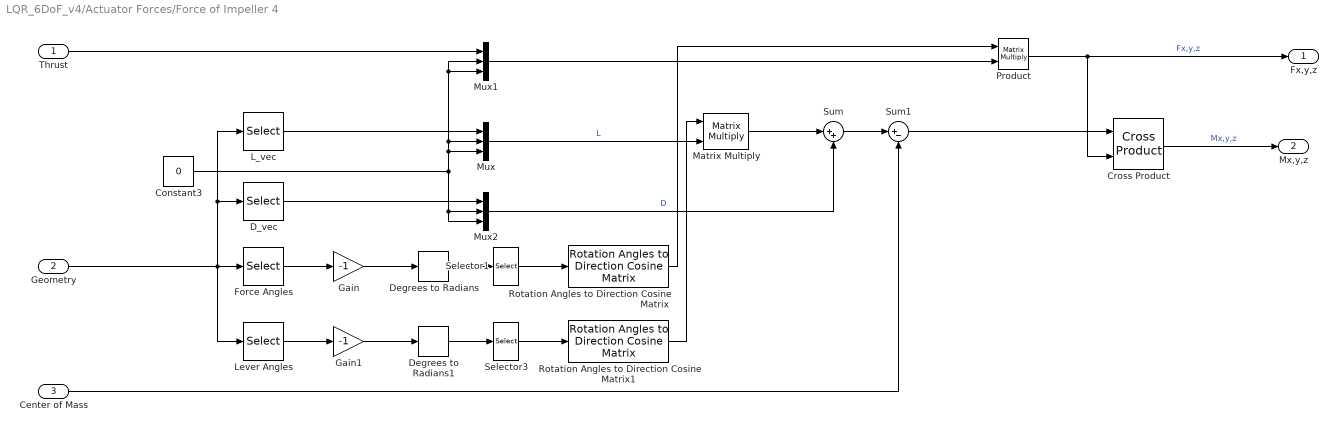
== system LQR_6DoF_v4/Actuator Forces/Force of Impeller 4 ==
  Thrust : Inport
  Geometry : Inport  Port=2
  Center of Mass : Inport  Port=3
  Constant3 : Constant  Value=0
  Cross Product : matrix_library/Cross Product
  D_vec : Selector  InputPortWidth=9  IndexOptions=Index vector (dialog)  Indices=[2]  OutputSizes=1
  Degrees to Radians : simulink_extras/Transformations/Degrees to Radians
  Degrees to Radians1 : simulink_extras/Transformations/Degrees to Radians
  Force Angles : Selector  InputPortWidth=9  IndexOptions=Index vector (dialog)  Indices=[4:6]  OutputSizes=1
  Gain : Gain  Gain=-1
  Gain1 : Gain  Gain=-1
  L_vec : Selector  InputPortWidth=9  IndexOptions=Index vector (dialog)  Indices=[1]  OutputSizes=1
  Lever Angles : Selector  InputPortWidth=9  IndexOptions=Index vector (dialog)  Indices=[7:9]  OutputSizes=1
  Matrix Multiply : Product  Multiplication=Matrix(*)
  Mux : Mux  Inputs=3
  Mux1 : Mux  Inputs=3
  Mux2 : Mux  Inputs=3
  Product : Product  Multiplication=Matrix(*)
  Rotation Angles to Direction Cosine Matrix : sharedtransform/Rotation Angles to Direction Cosine Matrix  rotationOrder=ZYX  aMode=aMode
  Rotation Angles to Direction Cosine Matrix1 : sharedtransform/Rotation Angles to Direction Cosine Matrix  rotationOrder=ZYX  aMode=aMode
  Selector1 : Selector  InputPortWidth=3  IndexOptions=Index vector (dialog)  Indices=[2 3 1]  OutputSizes=1
  Selector3 : Selector  InputPortWidth=3  IndexOptions=Index vector (dialog)  Indices=[2 3 1]  OutputSizes=1
  Sum : Sum  Inputs=|++
  Sum1 : Sum  Inputs=|+-
  Fx,y,z : Outport
  Mx,y,z : Outport  Port=2
  wires:
  Product/1 -> Fx,y,z/1, Cross Product/2  "Fx,y,z"
  Rotation Angles to Direction Cosine Matrix1/1 -> Matrix Multiply/1
  Constant3/1 -> Mux2/3, Mux2/2, Mux/3, Mux1/3, Mux1/2, Mux/2
  Degrees to Radians/1 -> Selector1/1
  Mux2/1 -> Sum/2  "D"
  Cross Product/1 -> Mx,y,z/1  "Mx,y,z"
  Mux1/1 -> Product/2
  Rotation Angles to Direction Cosine Matrix/1 -> Product/1
  Sum1/1 -> Cross Product/1
  Geometry/1 -> Force Angles/1, Lever Angles/1, D_vec/1, L_vec/1
  Sum/1 -> Sum1/1
  Degrees to Radians1/1 -> Selector3/1
  L_vec/1 -> Mux/1
  D_vec/1 -> Mux2/1
  Selector3/1 -> Rotation Angles to Direction Cosine Matrix1/1
  Force Angles/1 -> Gain/1
  Selector1/1 -> Rotation Angles to Direction Cosine Matrix/1
  Mux/1 -> Matrix Multiply/2  "L"
  Matrix Multiply/1 -> Sum/1
  Lever Angles/1 -> Gain1/1
  Thrust/1 -> Mux1/1
  Center of Mass/1 -> Sum1/2
  Gain/1 -> Degrees to Radians/1
  Gain1/1 -> Degrees to Radians1/1

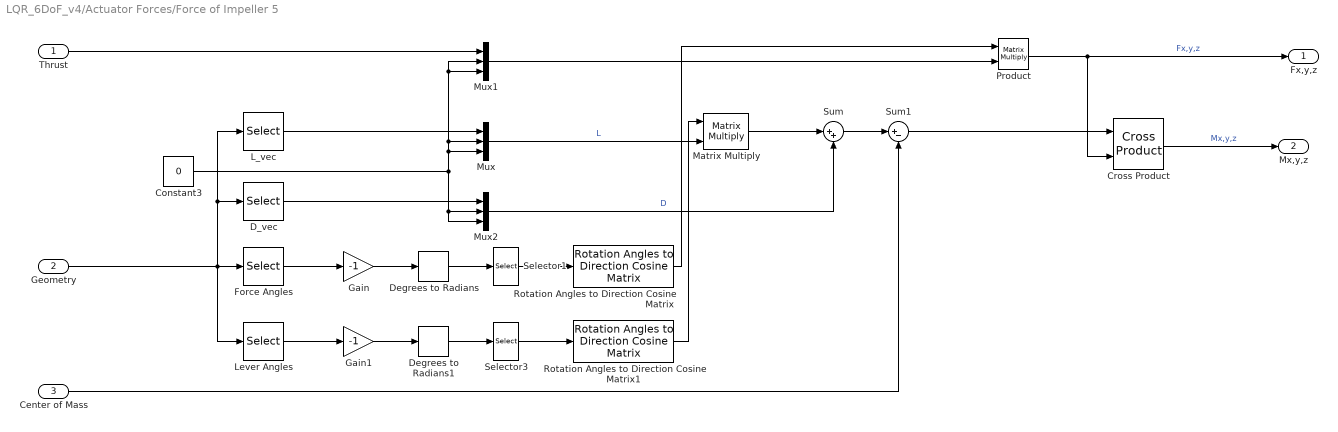
== system LQR_6DoF_v4/Actuator Forces/Force of Impeller 5 ==
  Thrust : Inport
  Geometry : Inport  Port=2
  Center of Mass : Inport  Port=3
  Constant3 : Constant  Value=0
  Cross Product : matrix_library/Cross Product
  D_vec : Selector  InputPortWidth=9  IndexOptions=Index vector (dialog)  Indices=[2]  OutputSizes=1
  Degrees to Radians : simulink_extras/Transformations/Degrees to Radians
  Degrees to Radians1 : simulink_extras/Transformations/Degrees to Radians
  Force Angles : Selector  InputPortWidth=9  IndexOptions=Index vector (dialog)  Indices=[4:6]  OutputSizes=1
  Gain : Gain  Gain=-1
  Gain1 : Gain  Gain=-1
  L_vec : Selector  InputPortWidth=9  IndexOptions=Index vector (dialog)  Indices=[1]  OutputSizes=1
  Lever Angles : Selector  InputPortWidth=9  IndexOptions=Index vector (dialog)  Indices=[7:9]  OutputSizes=1
  Matrix Multiply : Product  Multiplication=Matrix(*)
  Mux : Mux  Inputs=3
  Mux1 : Mux  Inputs=3
  Mux2 : Mux  Inputs=3
  Product : Product  Multiplication=Matrix(*)
  Rotation Angles to Direction Cosine Matrix : sharedtransform/Rotation Angles to Direction Cosine Matrix  rotationOrder=ZYX  aMode=aMode
  Rotation Angles to Direction Cosine Matrix1 : sharedtransform/Rotation Angles to Direction Cosine Matrix  rotationOrder=ZYX  aMode=aMode
  Selector1 : Selector  InputPortWidth=3  IndexOptions=Index vector (dialog)  Indices=[2 3 1]  OutputSizes=1
  Selector3 : Selector  InputPortWidth=3  IndexOptions=Index vector (dialog)  Indices=[2 3 1]  OutputSizes=1
  Sum : Sum  Inputs=|++
  Sum1 : Sum  Inputs=|+-
  Fx,y,z : Outport
  Mx,y,z : Outport  Port=2
  wires:
  Product/1 -> Fx,y,z/1, Cross Product/2  "Fx,y,z"
  Rotation Angles to Direction Cosine Matrix1/1 -> Matrix Multiply/1
  Constant3/1 -> Mux2/3, Mux2/2, Mux/3, Mux1/3, Mux1/2, Mux/2
  Degrees to Radians/1 -> Selector1/1
  Mux2/1 -> Sum/2  "D"
  Cross Product/1 -> Mx,y,z/1  "Mx,y,z"
  Mux1/1 -> Product/2
  Rotation Angles to Direction Cosine Matrix/1 -> Product/1
  Sum1/1 -> Cross Product/1
  Geometry/1 -> Force Angles/1, Lever Angles/1, D_vec/1, L_vec/1
  Sum/1 -> Sum1/1
  Degrees to Radians1/1 -> Selector3/1
  L_vec/1 -> Mux/1
  D_vec/1 -> Mux2/1
  Selector3/1 -> Rotation Angles to Direction Cosine Matrix1/1
  Force Angles/1 -> Gain/1
  Selector1/1 -> Rotation Angles to Direction Cosine Matrix/1
  Mux/1 -> Matrix Multiply/2  "L"
  Matrix Multiply/1 -> Sum/1
  Lever Angles/1 -> Gain1/1
  Thrust/1 -> Mux1/1
  Center of Mass/1 -> Sum1/2
  Gain/1 -> Degrees to Radians/1
  Gain1/1 -> Degrees to Radians1/1

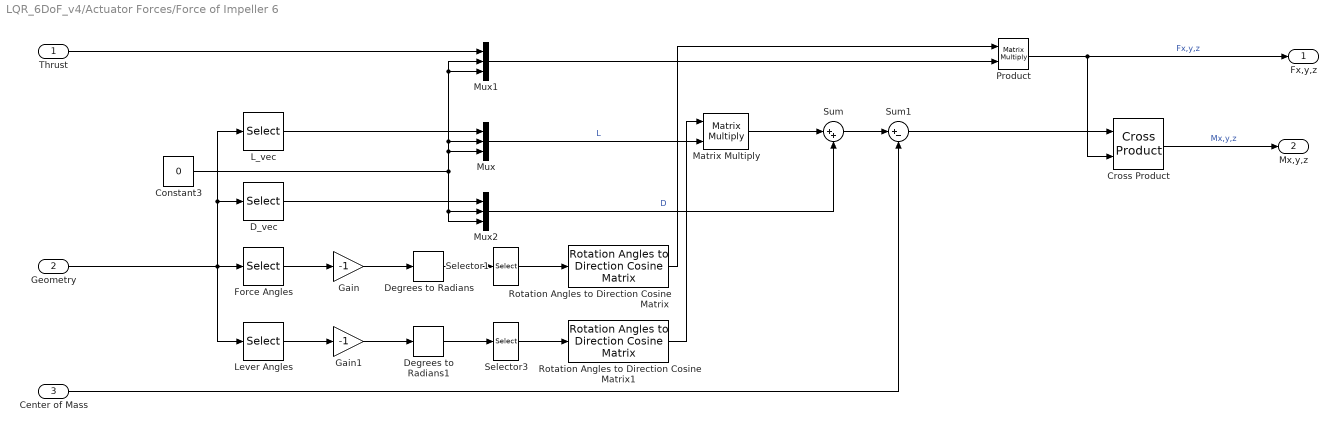
== system LQR_6DoF_v4/Actuator Forces/Force of Impeller 6 ==
  Thrust : Inport
  Geometry : Inport  Port=2
  Center of Mass : Inport  Port=3
  Constant3 : Constant  Value=0
  Cross Product : matrix_library/Cross Product
  D_vec : Selector  InputPortWidth=9  IndexOptions=Index vector (dialog)  Indices=[2]  OutputSizes=1
  Degrees to Radians : simulink_extras/Transformations/Degrees to Radians
  Degrees to Radians1 : simulink_extras/Transformations/Degrees to Radians
  Force Angles : Selector  InputPortWidth=9  IndexOptions=Index vector (dialog)  Indices=[4:6]  OutputSizes=1
  Gain : Gain  Gain=-1
  Gain1 : Gain  Gain=-1
  L_vec : Selector  InputPortWidth=9  IndexOptions=Index vector (dialog)  Indices=[1]  OutputSizes=1
  Lever Angles : Selector  InputPortWidth=9  IndexOptions=Index vector (dialog)  Indices=[7:9]  OutputSizes=1
  Matrix Multiply : Product  Multiplication=Matrix(*)
  Mux : Mux  Inputs=3
  Mux1 : Mux  Inputs=3
  Mux2 : Mux  Inputs=3
  Product : Product  Multiplication=Matrix(*)
  Rotation Angles to Direction Cosine Matrix : sharedtransform/Rotation Angles to Direction Cosine Matrix  rotationOrder=ZYX  aMode=aMode
  Rotation Angles to Direction Cosine Matrix1 : sharedtransform/Rotation Angles to Direction Cosine Matrix  rotationOrder=ZYX  aMode=aMode
  Selector1 : Selector  InputPortWidth=3  IndexOptions=Index vector (dialog)  Indices=[2 3 1]  OutputSizes=1
  Selector3 : Selector  InputPortWidth=3  IndexOptions=Index vector (dialog)  Indices=[2 3 1]  OutputSizes=1
  Sum : Sum  Inputs=|++
  Sum1 : Sum  Inputs=|+-
  Fx,y,z : Outport
  Mx,y,z : Outport  Port=2
  wires:
  Product/1 -> Fx,y,z/1, Cross Product/2  "Fx,y,z"
  Rotation Angles to Direction Cosine Matrix1/1 -> Matrix Multiply/1
  Constant3/1 -> Mux2/3, Mux2/2, Mux/3, Mux1/3, Mux1/2, Mux/2
  Degrees to Radians/1 -> Selector1/1
  Mux2/1 -> Sum/2  "D"
  Cross Product/1 -> Mx,y,z/1  "Mx,y,z"
  Mux1/1 -> Product/2
  Rotation Angles to Direction Cosine Matrix/1 -> Product/1
  Sum1/1 -> Cross Product/1
  Geometry/1 -> Force Angles/1, Lever Angles/1, D_vec/1, L_vec/1
  Sum/1 -> Sum1/1
  Degrees to Radians1/1 -> Selector3/1
  L_vec/1 -> Mux/1
  D_vec/1 -> Mux2/1
  Selector3/1 -> Rotation Angles to Direction Cosine Matrix1/1
  Force Angles/1 -> Gain/1
  Selector1/1 -> Rotation Angles to Direction Cosine Matrix/1
  Mux/1 -> Matrix Multiply/2  "L"
  Matrix Multiply/1 -> Sum/1
  Lever Angles/1 -> Gain1/1
  Thrust/1 -> Mux1/1
  Center of Mass/1 -> Sum1/2
  Gain/1 -> Degrees to Radians/1
  Gain1/1 -> Degrees to Radians1/1

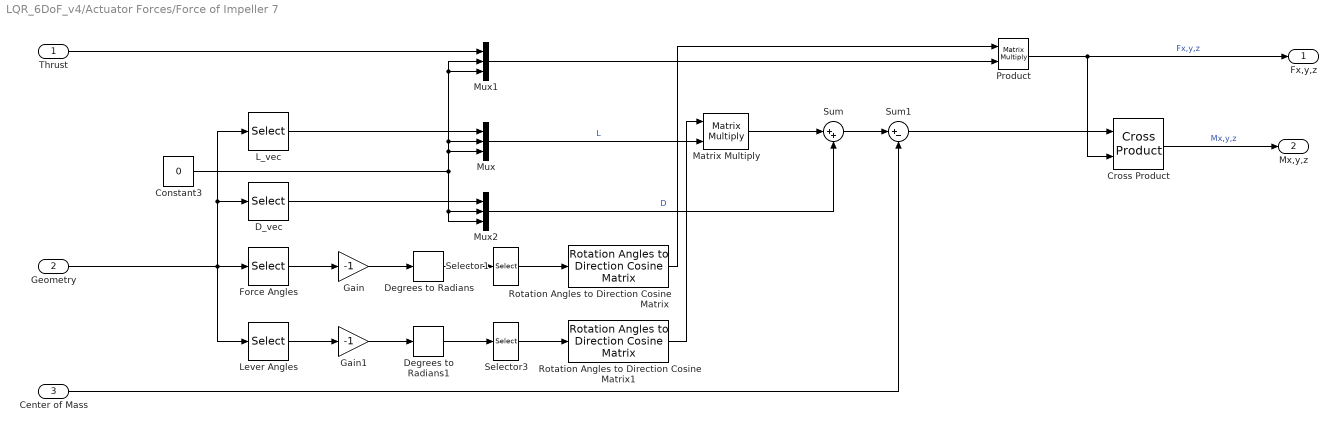
== system LQR_6DoF_v4/Actuator Forces/Force of Impeller 7 ==
  Thrust : Inport
  Geometry : Inport  Port=2
  Center of Mass : Inport  Port=3
  Constant3 : Constant  Value=0
  Cross Product : matrix_library/Cross Product
  D_vec : Selector  InputPortWidth=9  IndexOptions=Index vector (dialog)  Indices=[2]  OutputSizes=1
  Degrees to Radians : simulink_extras/Transformations/Degrees to Radians
  Degrees to Radians1 : simulink_extras/Transformations/Degrees to Radians
  Force Angles : Selector  InputPortWidth=9  IndexOptions=Index vector (dialog)  Indices=[4:6]  OutputSizes=1
  Gain : Gain  Gain=-1
  Gain1 : Gain  Gain=-1
  L_vec : Selector  InputPortWidth=9  IndexOptions=Index vector (dialog)  Indices=[1]  OutputSizes=1
  Lever Angles : Selector  InputPortWidth=9  IndexOptions=Index vector (dialog)  Indices=[7:9]  OutputSizes=1
  Matrix Multiply : Product  Multiplication=Matrix(*)
  Mux : Mux  Inputs=3
  Mux1 : Mux  Inputs=3
  Mux2 : Mux  Inputs=3
  Product : Product  Multiplication=Matrix(*)
  Rotation Angles to Direction Cosine Matrix : sharedtransform/Rotation Angles to Direction Cosine Matrix  rotationOrder=ZYX  aMode=aMode
  Rotation Angles to Direction Cosine Matrix1 : sharedtransform/Rotation Angles to Direction Cosine Matrix  rotationOrder=ZYX  aMode=aMode
  Selector1 : Selector  InputPortWidth=3  IndexOptions=Index vector (dialog)  Indices=[2 3 1]  OutputSizes=1
  Selector3 : Selector  InputPortWidth=3  IndexOptions=Index vector (dialog)  Indices=[2 3 1]  OutputSizes=1
  Sum : Sum  Inputs=|++
  Sum1 : Sum  Inputs=|+-
  Fx,y,z : Outport
  Mx,y,z : Outport  Port=2
  wires:
  Product/1 -> Fx,y,z/1, Cross Product/2  "Fx,y,z"
  Rotation Angles to Direction Cosine Matrix1/1 -> Matrix Multiply/1
  Constant3/1 -> Mux2/3, Mux2/2, Mux/3, Mux1/3, Mux1/2, Mux/2
  Degrees to Radians/1 -> Selector1/1
  Mux2/1 -> Sum/2  "D"
  Cross Product/1 -> Mx,y,z/1  "Mx,y,z"
  Mux1/1 -> Product/2
  Rotation Angles to Direction Cosine Matrix/1 -> Product/1
  Sum1/1 -> Cross Product/1
  Geometry/1 -> Force Angles/1, Lever Angles/1, D_vec/1, L_vec/1
  Sum/1 -> Sum1/1
  Degrees to Radians1/1 -> Selector3/1
  L_vec/1 -> Mux/1
  D_vec/1 -> Mux2/1
  Selector3/1 -> Rotation Angles to Direction Cosine Matrix1/1
  Force Angles/1 -> Gain/1
  Selector1/1 -> Rotation Angles to Direction Cosine Matrix/1
  Mux/1 -> Matrix Multiply/2  "L"
  Matrix Multiply/1 -> Sum/1
  Lever Angles/1 -> Gain1/1
  Thrust/1 -> Mux1/1
  Center of Mass/1 -> Sum1/2
  Gain/1 -> Degrees to Radians/1
  Gain1/1 -> Degrees to Radians1/1

== system LQR_6DoF_v4/Actuator Forces/Force of Impeller 8 ==
  Thrust : Inport
  Geometry : Inport  Port=2
  Center of Mass : Inport  Port=3
  Constant3 : Constant  Value=0
  Cross Product : matrix_library/Cross Product
  D_vec : Selector  InputPortWidth=9  IndexOptions=Index vector (dialog)  Indices=[2]  OutputSizes=1
  Degrees to Radians : simulink_extras/Transformations/Degrees to Radians
  Degrees to Radians1 : simulink_extras/Transformations/Degrees to Radians
  Force Angles : Selector  InputPortWidth=9  IndexOptions=Index vector (dialog)  Indices=[4:6]  OutputSizes=1
  Gain : Gain  Gain=-1
  Gain1 : Gain  Gain=-1
  L_vec : Selector  InputPortWidth=9  IndexOptions=Index vector (dialog)  Indices=[1]  OutputSizes=1
  Lever Angles : Selector  InputPortWidth=9  IndexOptions=Index vector (dialog)  Indices=[7:9]  OutputSizes=1
  Matrix Multiply : Product  Multiplication=Matrix(*)
  Mux : Mux  Inputs=3
  Mux1 : Mux  Inputs=3
  Mux2 : Mux  Inputs=3
  Product : Product  Multiplication=Matrix(*)
  Rotation Angles to Direction Cosine Matrix : sharedtransform/Rotation Angles to Direction Cosine Matrix  rotationOrder=ZYX  aMode=aMode
  Rotation Angles to Direction Cosine Matrix1 : sharedtransform/Rotation Angles to Direction Cosine Matrix  rotationOrder=ZYX  aMode=aMode
  Selector1 : Selector  InputPortWidth=3  IndexOptions=Index vector (dialog)  Indices=[2 3 1]  OutputSizes=1
  Selector3 : Selector  InputPortWidth=3  IndexOptions=Index vector (dialog)  Indices=[2 3 1]  OutputSizes=1
  Sum : Sum  Inputs=|++
  Sum1 : Sum  Inputs=|+-
  Fx,y,z : Outport
  Mx,y,z : Outport  Port=2
  wires:
  Product/1 -> Fx,y,z/1, Cross Product/2  "Fx,y,z"
  Rotation Angles to Direction Cosine Matrix1/1 -> Matrix Multiply/1
  Constant3/1 -> Mux2/3, Mux2/2, Mux/3, Mux1/3, Mux1/2, Mux/2
  Degrees to Radians/1 -> Selector1/1
  Mux2/1 -> Sum/2  "D"
  Cross Product/1 -> Mx,y,z/1  "Mx,y,z"
  Mux1/1 -> Product/2
  Rotation Angles to Direction Cosine Matrix/1 -> Product/1
  Sum1/1 -> Cross Product/1
  Geometry/1 -> Force Angles/1, Lever Angles/1, D_vec/1, L_vec/1
  Sum/1 -> Sum1/1
  Degrees to Radians1/1 -> Selector3/1
  L_vec/1 -> Mux/1
  D_vec/1 -> Mux2/1
  Selector3/1 -> Rotation Angles to Direction Cosine Matrix1/1
  Force Angles/1 -> Gain/1
  Selector1/1 -> Rotation Angles to Direction Cosine Matrix/1
  Mux/1 -> Matrix Multiply/2  "L"
  Matrix Multiply/1 -> Sum/1
  Lever Angles/1 -> Gain1/1
  Thrust/1 -> Mux1/1
  Center of Mass/1 -> Sum1/2
  Gain/1 -> Degrees to Radians/1
  Gain1/1 -> Degrees to Radians1/1

== system LQR_6DoF_v4/Actuator Forces/Force of Impeller 9 ==
  Thrust : Inport
  Geometry : Inport  Port=2
  Center of Mass : Inport  Port=3
  Constant3 : Constant  Value=0
  Cross Product : matrix_library/Cross Product
  D_vec : Selector  InputPortWidth=9  IndexOptions=Index vector (dialog)  Indices=[2]  OutputSizes=1
  Degrees to Radians : simulink_extras/Transformations/Degrees to Radians
  Degrees to Radians1 : simulink_extras/Transformations/Degrees to Radians
  Force Angles : Selector  InputPortWidth=9  IndexOptions=Index vector (dialog)  Indices=[4:6]  OutputSizes=1
  Gain : Gain  Gain=-1
  Gain1 : Gain  Gain=-1
  L_vec : Selector  InputPortWidth=9  IndexOptions=Index vector (dialog)  Indices=[1]  OutputSizes=1
  Lever Angles : Selector  InputPortWidth=9  IndexOptions=Index vector (dialog)  Indices=[7:9]  OutputSizes=1
  Matrix Multiply : Product  Multiplication=Matrix(*)
  Mux : Mux  Inputs=3
  Mux1 : Mux  Inputs=3
  Mux2 : Mux  Inputs=3
  Product : Product  Multiplication=Matrix(*)
  Rotation Angles to Direction Cosine Matrix : sharedtransform/Rotation Angles to Direction Cosine Matrix  rotationOrder=ZYX  aMode=aMode
  Rotation Angles to Direction Cosine Matrix1 : sharedtransform/Rotation Angles to Direction Cosine Matrix  rotationOrder=ZYX  aMode=aMode
  Selector1 : Selector  InputPortWidth=3  IndexOptions=Index vector (dialog)  Indices=[2 3 1]  OutputSizes=1
  Selector3 : Selector  InputPortWidth=3  IndexOptions=Index vector (dialog)  Indices=[2 3 1]  OutputSizes=1
  Sum : Sum  Inputs=|++
  Sum1 : Sum  Inputs=|+-
  Fx,y,z : Outport
  Mx,y,z : Outport  Port=2
  wires:
  Product/1 -> Fx,y,z/1, Cross Product/2  "Fx,y,z"
  Rotation Angles to Direction Cosine Matrix1/1 -> Matrix Multiply/1
  Constant3/1 -> Mux2/3, Mux2/2, Mux/3, Mux1/3, Mux1/2, Mux/2
  Degrees to Radians/1 -> Selector1/1
  Mux2/1 -> Sum/2  "D"
  Cross Product/1 -> Mx,y,z/1  "Mx,y,z"
  Mux1/1 -> Product/2
  Rotation Angles to Direction Cosine Matrix/1 -> Product/1
  Sum1/1 -> Cross Product/1
  Geometry/1 -> Force Angles/1, Lever Angles/1, D_vec/1, L_vec/1
  Sum/1 -> Sum1/1
  Degrees to Radians1/1 -> Selector3/1
  L_vec/1 -> Mux/1
  D_vec/1 -> Mux2/1
  Selector3/1 -> Rotation Angles to Direction Cosine Matrix1/1
  Force Angles/1 -> Gain/1
  Selector1/1 -> Rotation Angles to Direction Cosine Matrix/1
  Mux/1 -> Matrix Multiply/2  "L"
  Matrix Multiply/1 -> Sum/1
  Lever Angles/1 -> Gain1/1
  Thrust/1 -> Mux1/1
  Center of Mass/1 -> Sum1/2
  Gain/1 -> Degrees to Radians/1
  Gain1/1 -> Degrees to Radians1/1

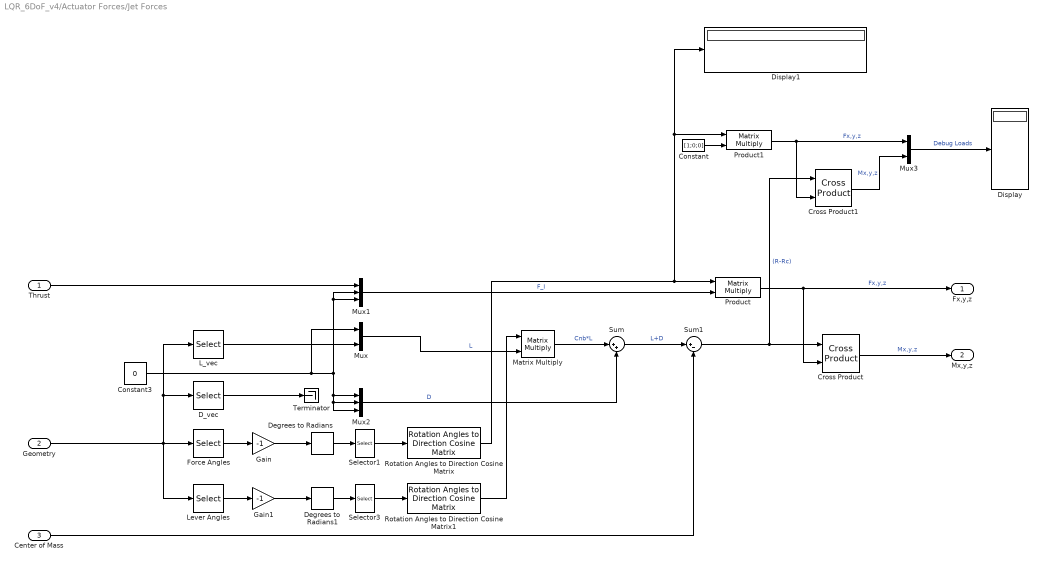
== system LQR_6DoF_v4/Actuator Forces/Jet Forces ==
  Thrust : Inport
  Geometry : Inport  Port=2
  Center of Mass : Inport  Port=3
  Constant : Constant  Value=[1;0;0]
  Constant3 : Constant  Value=0
  Cross Product : matrix_library/Cross Product
  Cross Product1 : matrix_library/Cross Product
  D_vec : Selector  InputPortWidth=9  IndexOptions=Index vector (dialog)  Indices=[2]  OutputSizes=1
  Degrees to Radians : simulink_extras/Transformations/Degrees to Radians
  Degrees to Radians1 : simulink_extras/Transformations/Degrees to Radians
  Display : Display
  Display1 : Display
  Force Angles : Selector  InputPortWidth=9  IndexOptions=Index vector (dialog)  Indices=[4:6]  OutputSizes=1
  Gain : Gain  Gain=-1
  Gain1 : Gain  Gain=-1
  L_vec : Selector  InputPortWidth=9  IndexOptions=Index vector (dialog)  Indices=[2 3]  OutputSizes=1
  Lever Angles : Selector  InputPortWidth=9  IndexOptions=Index vector (dialog)  Indices=[7:9]  OutputSizes=1
  Matrix Multiply : Product  Multiplication=Matrix(*)
  Mux : Mux  Inputs=2
  Mux1 : Mux  Inputs=3
  Mux2 : Mux  Inputs=3
  Mux3 : Mux  Inputs=2
  Product : Product  Multiplication=Matrix(*)
  Product1 : Product  Multiplication=Matrix(*)
  Rotation Angles to Direction Cosine Matrix : sharedtransform/Rotation Angles to Direction Cosine Matrix  rotationOrder=ZYX  aMode=aMode
  Rotation Angles to Direction Cosine Matrix1 : sharedtransform/Rotation Angles to Direction Cosine Matrix  rotationOrder=ZYX  aMode=aMode
  Selector1 : Selector  InputPortWidth=3  IndexOptions=Index vector (dialog)  Indices=[2 3 1]  OutputSizes=1
  Selector3 : Selector  InputPortWidth=3  IndexOptions=Index vector (dialog)  Indices=[2 3 1]  OutputSizes=1
  Sum : Sum  Inputs=|++
  Sum1 : Sum  Inputs=|+-
  Terminator : Terminator
  Fx,y,z : Outport
  Mx,y,z : Outport  Port=2
  wires:
  Product/1 -> Fx,y,z/1, Cross Product/2  "Fx,y,z"
  Rotation Angles to Direction Cosine Matrix1/1 -> Matrix Multiply/1
  Constant3/1 -> Mux2/1, Mux2/3, Mux2/2, Mux1/3, Mux1/2, Mux/1
  Degrees to Radians/1 -> Selector1/1
  Mux2/1 -> Sum/2  "D"
  Cross Product/1 -> Mx,y,z/1  "Mx,y,z"
  Mux1/1 -> Product/2  "F_I"
  Rotation Angles to Direction Cosine Matrix/1 -> Display1/1, Product1/1, Product/1
  Sum1/1 -> Cross Product/1, Cross Product1/1  "(R-Rc)"
  Geometry/1 -> Force Angles/1, Lever Angles/1, D_vec/1, L_vec/1
  Sum/1 -> Sum1/1  "L+D"
  Degrees to Radians1/1 -> Selector3/1
  L_vec/1 -> Mux/2
  D_vec/1 -> Terminator/1
  Selector3/1 -> Rotation Angles to Direction Cosine Matrix1/1
  Force Angles/1 -> Gain/1
  Selector1/1 -> Rotation Angles to Direction Cosine Matrix/1
  Mux/1 -> Matrix Multiply/2  "L"
  Matrix Multiply/1 -> Sum/1  "Cnb*L"
  Lever Angles/1 -> Gain1/1
  Thrust/1 -> Mux1/1
  Center of Mass/1 -> Sum1/2
  Gain/1 -> Degrees to Radians/1
  Gain1/1 -> Degrees to Radians1/1
  Constant/1 -> Product1/2
  Product1/1 -> Mux3/1, Cross Product1/2  "Fx,y,z"
  Cross Product1/1 -> Mux3/2  "Mx,y,z"
  Mux3/1 -> Display/1  "Debug Loads"

== system LQR_6DoF_v4/Earth2NED/Euler2DCM ==
  "Roll, Pitch, Yaw" : Inport
  "Pitch, Yaw, Roll" : Selector  InputPortWidth=3  IndexOptions=Index vector (dialog)  Indices=[2 3 1]  OutputSizes=1
  Quaternions to Direction Cosine Matrix : sharedtransform/Quaternions to  Direction Cosine Matrix  aMode=aMode
  Rotation Angles to Quaternions : sharedtransform/Rotation Angles to Quaternions  rotationOrder=ZYX  aMode=aMode
  DCM : Outport
  wires:
  "Roll, Pitch, Yaw"/1 -> "Pitch, Yaw, Roll"/1
  "Pitch, Yaw, Roll"/1 -> Rotation Angles to Quaternions/1
  Rotation Angles to Quaternions/1 -> Quaternions to Direction Cosine Matrix/1
  Quaternions to Direction Cosine Matrix/1 -> DCM/1
